simulink model "Lambda_4"  (R2016b)
settings: Solver=FixedStepAuto  StartTime=0.0  StopTime=tF  FixedStep=0.01  RelTol=1e-3
values from neighbouring files (symbols this model uses):
  K = 0.2*sgn    [parameters.m]    (also in vec_s1.mat = 0.2)
  K_dth = 0.2*sgn    [parameters.m]    (also in vec_s1.mat = 0.05)
  M_d = 200*sgn    [parameters.m]    (also in vec_s1.mat = 200)
  N = 3    [parameters.m]    (also in vec_s1.mat)
  R_0 = Vc*tF    [Proj_2_4.m]
  rho_v = 15    [parameters.m]    (also in vec_s1.mat)
  T_m = 120    [parameters.m]    (also in vec_s1.mat)
  tau = 0.05    [parameters.m]    (also in vec_s1.mat)
  tF = 1.5    [Controllers_Design.m]    (also in Proj_1.m; Proj_2.m; Proj_2_4.m = 4; vec_s1.mat)
  Vc = 1250    [parameters.m]    (also in vec_s1.mat)
undefined symbols (not defined in the file or in its folder): R0
settings Model: Creator=Daniel  LastModifiedBy=Daniel

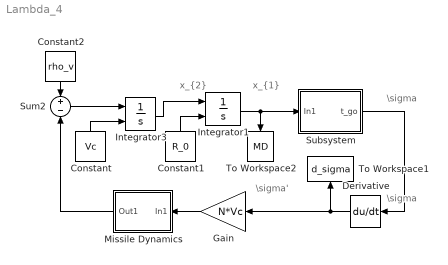
== system Lambda_4 ==
  note: x_{2}
  note: \sigma
  note: \sigma'
  note: x_{1}
  note: \sigma
  Constant : Constant  Value=Vc
  Constant1 : Constant  Value=R_0
  Constant2 : Constant  Value=rho_v
  Derivative : Derivative
  Gain : Gain  Gain=N*Vc
  Integrator1 : Integrator  InitialConditionSource=external  InitialCondition=Vc
  Integrator3 : Integrator  InitialConditionSource=external  InitialCondition=R0
  Missile Dynamics : Subsystem
      mask Display: image('Gm_s.PNG');
  Subsystem : Subsystem
      mask Display: image('Vc_tf.png');
  Sum2 : Sum  Inputs=+|-
  To Workspace1 : ToWorkspace  VariableName=d_sigma  SaveFormat=Timeseries  SampleTime=-1
  To Workspace2 : ToWorkspace  VariableName=MD  SaveFormat=Timeseries  SampleTime=-1
  wires:
  Missile Dynamics/1(Out1) -> Sum2/2
  Integrator1/1 -> Subsystem/1(In1), To Workspace2/1
  Integrator3/1 -> Integrator1/1
  Constant1/1 -> Integrator1/2
  Constant/1 -> Integrator3/2
  Gain/1 -> Missile Dynamics/1(In1)
  Sum2/1 -> Integrator3/1
  Constant2/1 -> Sum2/1
  Derivative/1 -> Gain/1, To Workspace1/1
  Subsystem/1(t_go) -> Derivative/1

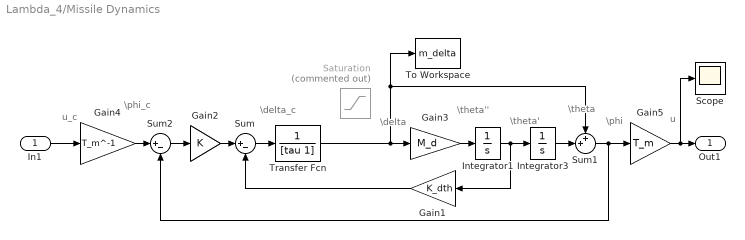
== system Lambda_4/Missile Dynamics ==
  note: \theta'
  note: \theta''
  note: \theta
  note: \delta
  note: \delta_c
  note: \phi_c
  note: \phi
  note: u
  note: u_c
  In1 : Inport
  Gain1 : Gain  Gain=K_dth
  Gain2 : Gain  Gain=K
  Gain3 : Gain  Gain=M_d
  Gain4 : Gain  Gain=T_m^-1
  Gain5 : Gain  Gain=T_m
  Integrator1 : Integrator
  Integrator3 : Integrator
  Saturation : Saturate  Commented=on  UpperLimit=0.5237  LowerLimit=-0.5237
  Scope : Scope
  Sum : Sum  Inputs=|+-
  Sum1 : Sum  Inputs=++|
  Sum2 : Sum  Inputs=|+-
  To Workspace : ToWorkspace  VariableName=m_delta  SaveFormat=Timeseries  SampleTime=-1
  Transfer Fcn : TransferFcn  Denominator=[tau 1]
  Out1 : Outport
  wires:
  Gain1/1 -> Sum/2
  Sum/1 -> Transfer Fcn/1
  Gain2/1 -> Sum/1
  Sum1/1 -> Sum2/2, Gain5/1
  Gain3/1 -> Integrator1/1
  Integrator1/1 -> Integrator3/1, Gain1/1
  Integrator3/1 -> Sum1/2
  Sum2/1 -> Gain2/1
  Gain5/1 -> Scope/1, Out1/1
  In1/1 -> Gain4/1
  Gain4/1 -> Sum2/1
  Transfer Fcn/1 -> Sum1/1, To Workspace/1, Gain3/1

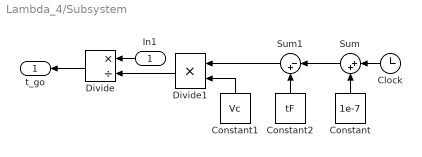
== system Lambda_4/Subsystem ==
  In1 : Inport
  Clock : Clock
  Constant : Constant  Value=1e-7
  Constant1 : Constant  Value=Vc
  Constant2 : Constant  Value=tF
  Divide : Product  Inputs=*/
  Divide1 : Product  Inputs=**
  Sum : Sum  Inputs=|++
  Sum1 : Sum  Inputs=|-+
  t_go : Outport
  wires:
  Sum/1 -> Sum1/1
  In1/1 -> Divide/1
  Divide/1 -> t_go/1
  Constant/1 -> Sum/2
  Clock/1 -> Sum/1
  Constant1/1 -> Divide1/2
  Constant2/1 -> Sum1/2
  Sum1/1 -> Divide1/1
  Divide1/1 -> Divide/2
